simulink model "new_inkine_2020"  (R2022b)
settings: Solver=FixedStepAuto  StartTime=0.0  StopTime=250  FixedStep=0.001  RelTol=1e-3
PreLoadFcn:
  | parameters_new;
InitFcn:
  | parameters_new;
(part 1 of 3)
settings Model: Creator=Yubin  LastModifiedBy=峰
settings SolverCC: AlgebraicLoopSolver=TrustRegion
settings ConfigComp: PLC_OutputDir=D:\Documents\Visual Studio 2015\Projects  PLC_TargetIDE=twincat3  PLC_MultiTBSigbuilderTimeRange=off  PLC_FoldFBCallOutputVar=off  PLC_InlineEnumCastFunction=off

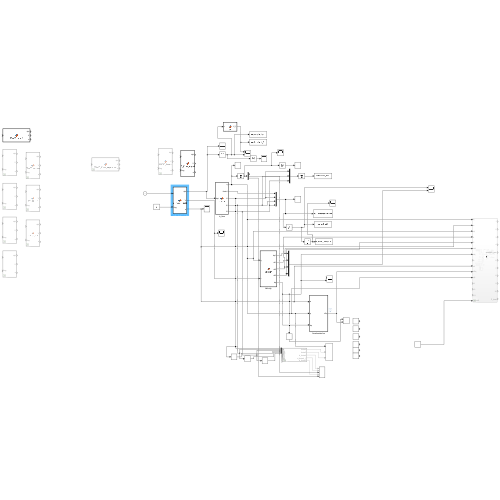
[thumbnail: Simulink's stored preview of the top-level diagram]
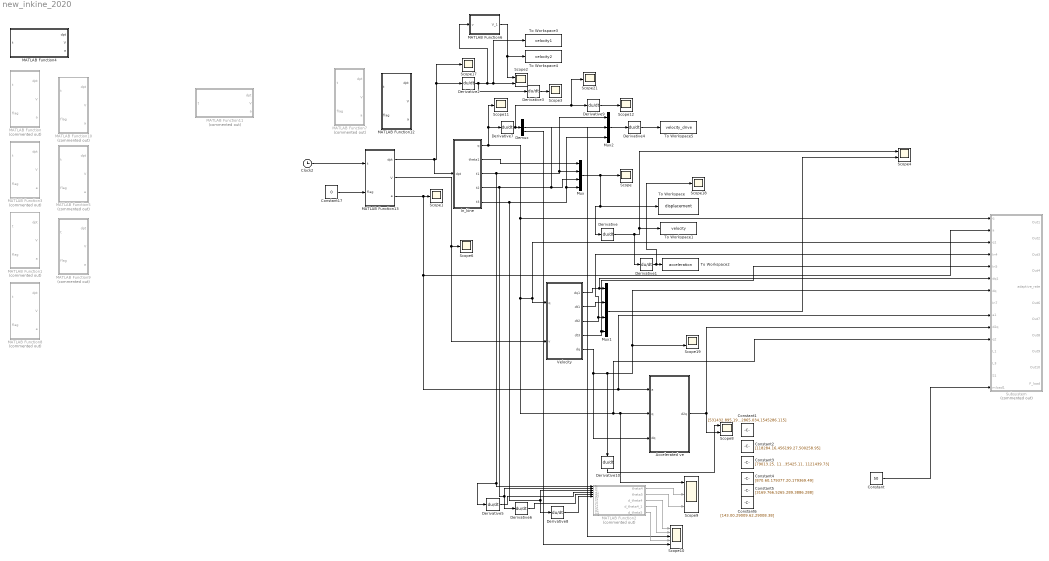
== system new_inkine_2020 ==
  Accelerated ve : MATLAB Function  TreatAsAtomicUnit=on
  Clock2 : Clock
      settings: Decimation=50
  Constant : Constant  Value=50
  Constant1 : Constant  Value=[531432.895,1962865.034,1545286.115]
  Constant17 : Constant  Value=0
  Constant2 : Constant  Value=[118284.16,456199.27,500258.95]
  Constant3 : Constant  Value=[79013.25, 1135425.11, 1121439.73]
  Constant4 : Constant  Value=[870.60,179377.20,179369.49]
  Constant5 : Constant  Value=[3169.766,5265.289,3886.288]
  Constant6 : Constant  Value=[143.00,29009.62,29008.38]
  Demux : Demux  Outputs=3
  Derivative{,1..10} (11 alike) : Derivative
  In_kine : MATLAB Function  TreatAsAtomicUnit=on
  MATLAB Function : MATLAB Function  Commented=on  TreatAsAtomicUnit=on
  MATLAB Function1 : MATLAB Function  Commented=on  TreatAsAtomicUnit=on
  MATLAB Function10 : MATLAB Function  Commented=on  TreatAsAtomicUnit=on
  MATLAB Function11 : MATLAB Function  Commented=on  TreatAsAtomicUnit=on
  MATLAB Function12 : MATLAB Function  TreatAsAtomicUnit=on
  MATLAB Function13 : MATLAB Function  TreatAsAtomicUnit=on
  MATLAB Function2 : MATLAB Function  Commented=on  TreatAsAtomicUnit=on
  MATLAB Function3 : MATLAB Function  Commented=on  TreatAsAtomicUnit=on
  MATLAB Function4 : MATLAB Function  TreatAsAtomicUnit=on
  MATLAB Function5 : MATLAB Function  Commented=on  TreatAsAtomicUnit=on
  MATLAB Function6 : MATLAB Function  TreatAsAtomicUnit=on
  MATLAB Function7 : MATLAB Function  Commented=on  TreatAsAtomicUnit=on
  MATLAB Function8 : MATLAB Function  Commented=on  TreatAsAtomicUnit=on
  MATLAB Function9 : MATLAB Function  Commented=on  TreatAsAtomicUnit=on
  Mux : Mux
  Mux1 : Mux
  Mux2 : Mux  Inputs=3
  Scope{,1,3,6,11..12,17..18,21} (9 alike) : Scope
  Scope10 : Scope  NumInputPorts=5
  Scope{2,4,8,19} (4 alike) : Scope  NumInputPorts=2
  Scope9 : Scope  NumInputPorts=3
  Subsystem : Subsystem  Commented=on
  To Workspace : ToWorkspace  VariableName=displacement  SaveFormat=Timeseries  SampleTime=-1
  To Workspace1 : ToWorkspace  VariableName=velocity  SaveFormat=Timeseries  SampleTime=-1
  To Workspace2 : ToWorkspace  VariableName=acceleration  SaveFormat=Timeseries  SampleTime=-1
  To Workspace3 : ToWorkspace  VariableName=velocity1  SampleTime=-1
      settings: Save2DSignal=2-D array (concatenate along first dimension)
  To Workspace4 : ToWorkspace  VariableName=velocity2  SampleTime=-1
      settings: Save2DSignal=2-D array (concatenate along first dimension)
  To Workspace5 : ToWorkspace  VariableName=velocity_drive  SampleTime=-1
      settings: Save2DSignal=2-D array (concatenate along first dimension)
  Velocity : MATLAB Function  TreatAsAtomicUnit=on
  wires:
  In_kine/2(theta1) -> Mux/1
  Clock2/1 -> MATLAB Function13/1(t)
  Derivative/1 -> Scope4/1, To Workspace1/1, Derivative1/1
  Derivative1/1 -> Scope18/1, To Workspace2/1
  MATLAB Function13/1(dpt) -> In_kine/1(dpt), Scope17/1, Derivative2/1
  Derivative3/1 -> Scope3/1
  MATLAB Function13/3(a) -> Subsystem/9(a1), Accelerated ve/1(a), Subsystem/2(a), Scope1/1
  Velocity/1(dq1) -> Subsystem/6(dq1), Mux1/1
  Velocity/2(dt1) -> Mux1/2
  Velocity/3(dt2) -> Mux1/3, Subsystem/4(In4)
  Velocity/4(dt3) -> Subsystem/5(In5), Mux1/4
  Mux1/1 -> Scope4/2
  MATLAB Function13/2(V) -> Velocity/2(v), Scope6/1
  Velocity/5(dq) -> Accelerated ve/3(dq), Subsystem/7(dq), Scope19/2, Derivative10/1
  Accelerated ve/1(d2q) -> Subsystem/10(d2q), Scope8/2
  MATLAB Function2/1(theta4) -> Scope9/2
  MATLAB Function2/2(theta5) -> Scope9/3
  MATLAB Function2/3(d_theta4) -> Scope10/1
  Demux/2 -> Scope10/3
  MATLAB Function2/5(d_theta5) -> Scope10/4
  Derivative7/1 -> Scope21/1, Derivative9/1, Demux/1
  Demux/3 -> Scope10/5
  MATLAB Function2/4(d_theta4_1) -> Scope10/2
  Derivative5/1 -> MATLAB Function2/4(dt1)
  In_kine/4(t2) -> Derivative6/1, MATLAB Function2/2(t2), Mux/3, Mux2/2
  In_kine/5(t3) -> Derivative8/1, MATLAB Function2/3(t3), Mux2/3, Mux/4
  Derivative6/1 -> MATLAB Function2/5(dt2)
  Derivative8/1 -> MATLAB Function2/6(dt3)
  Constant17/1 -> MATLAB Function13/2(flag)
  Derivative9/1 -> Scope12/1
  Mux/1 -> Scope/1, Derivative/1, To Workspace/1
  Derivative10/1 -> Scope8/1
  In_kine/1(q) -> Scope11/1, Derivative7/1, Subsystem/1(q), Velocity/1(q), Subsystem/3(q1), Subsystem/11(q2), Scope9/1, Accelerated ve/2(q)
  MATLAB Function6/1(V_1) -> To Workspace4/1, Scope2/1
  Constant/1 -> Subsystem/15(mload1)
  Derivative2/1 -> Derivative3/1, MATLAB Function6/1(v), Scope2/2, To Workspace3/1
  In_kine/3(t1) -> Derivative5/1, MATLAB Function2/1(t1), Mux/2, Mux2/1
  Mux2/1 -> Derivative4/1
  Derivative4/1 -> To Workspace5/1

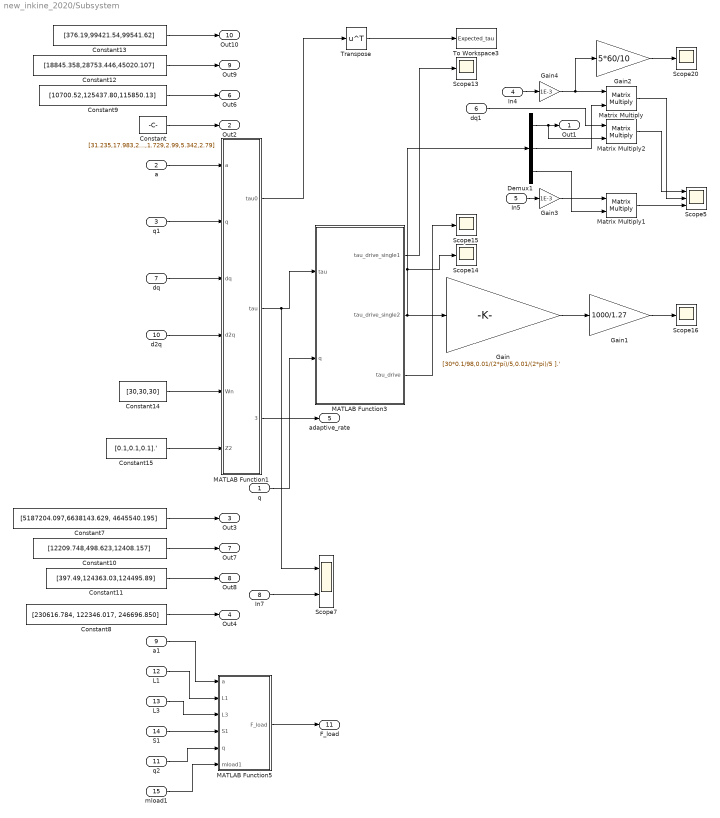
== system new_inkine_2020/Subsystem ==
  q : Inport
  a : Inport  Port=2
  q1 : Inport  Port=3
  In4 : Inport  Port=4
  In5 : Inport  Port=5
  dq1 : Inport  Port=6
  dq : Inport  Port=7
  In7 : Inport  Port=8
  a1 : Inport  Port=9
  d2q : Inport  Port=10
  q2 : Inport  Port=11
  L1 : Inport  Port=12
  L3 : Inport  Port=13
  S1 : Inport  Port=14
  mload1 : Inport  Port=15
  Constant : Constant  Value=[31.235,17.983,21.8,5.16,2.248,2.248,1.73,1.73,121.413,13.425,3.54,1.729,2.99,5.342,2.79]
  Constant10 : Constant  Value=[12209.748,498.623,12408.157]
  Constant11 : Constant  Value=[397.49,124363.03,124495.89]
  Constant12 : Constant  Value=[18845.358,28753.446,45020.107]
  Constant13 : Constant  Value=[376.19,99421.54,99541.62]
  Constant14 : Constant  Value=[30,30,30]
  Constant15 : Constant  Value=[0.1,0.1,0.1].'
  Constant7 : Constant  Value=[5187204.097,6638143.629, 4645540.195]
  Constant8 : Constant  Value=[230616.784, 122346.017, 246696.850]
  Constant9 : Constant  Value=[10700.52,125437.80,115850.13]
  Demux1 : Demux  Outputs=3
  Gain : Gain  Gain=[30*0.1/98,0.01/(2*pi)/5,0.01/(2*pi)/5 ].'
  Gain1 : Gain  Gain=1000/1.27
  Gain2 : Gain  Gain=5*60/10
  Gain3 : Gain  Gain=1E-3
  Gain4 : Gain  Gain=1E-3
  MATLAB Function1 : MATLAB Function  TreatAsAtomicUnit=on
  MATLAB Function3 : MATLAB Function  TreatAsAtomicUnit=on
  MATLAB Function5 : MATLAB Function  TreatAsAtomicUnit=on
  Matrix Multiply : Product  Multiplication=Matrix(*)
  Matrix Multiply1 : Product  Multiplication=Matrix(*)
  Matrix Multiply2 : Product  Multiplication=Matrix(*)
  Scope{13..16,20} (5 alike) : Scope
  Scope5 : Scope  NumInputPorts=3
  Scope7 : Scope  NumInputPorts=2
  To Workspace3 : ToWorkspace  VariableName=Expected_tau  SampleTime=-1
      settings: Save2DSignal=2-D array (concatenate along first dimension)
  Transpose : Math  Operator=transpose
  Out1 : Outport
  Out2 : Outport  Port=2
  Out3 : Outport  Port=3
  Out4 : Outport  Port=4
  adaptive_rate : Outport  Port=5
  Out6 : Outport  Port=6
  Out7 : Outport  Port=7
  Out8 : Outport  Port=8
  Out9 : Outport  Port=9
  Out10 : Outport  Port=10
  F_load : Outport  Port=11
  wires:
  Constant/1 -> Out2/1
  d2q/1 -> MATLAB Function1/4(d2q)
  Demux1/1 -> Matrix Multiply2/2, Out1/1
  L1/1 -> MATLAB Function5/2(L1)
  Constant13/1 -> Out10/1
  q1/1 -> MATLAB Function1/2(q)
  Constant9/1 -> Out6/1
  Constant12/1 -> Out9/1
  a/1 -> MATLAB Function1/1(a)
  dq/1 -> MATLAB Function1/3(dq)
  Constant15/1 -> MATLAB Function1/6(Z2)
  Constant14/1 -> MATLAB Function1/5(Wn)
  Constant7/1 -> Out3/1
  Constant10/1 -> Out7/1
  In7/1 -> Scope7/2
  Constant11/1 -> Out8/1
  In5/1 -> Gain3/1
  S1/1 -> MATLAB Function5/4(S1)
  Constant8/1 -> Out4/1
  q/1 -> MATLAB Function3/2(q)
  a1/1 -> MATLAB Function5/1(a)
  In4/1 -> Gain4/1
  L3/1 -> MATLAB Function5/3(L3)
  q2/1 -> MATLAB Function5/5(q)
  mload1/1 -> MATLAB Function5/6(mload1)
  MATLAB Function1/1(tau0) -> Transpose/1
  MATLAB Function1/2(tau) -> Scope7/1, MATLAB Function3/1(tau)
  Gain/1 -> Gain1/1
  MATLAB Function1/3(adaptive_rate) -> adaptive_rate/1
  MATLAB Function5/1(F_load) -> F_load/1
  Transpose/1 -> To Workspace3/1
  MATLAB Function3/3(tau_drive) -> Scope15/1
  MATLAB Function3/1(tau_drive_single1) -> Scope13/1
  MATLAB Function3/2(tau_drive_single2) -> Scope14/1, Demux1/1, Gain/1
  Demux1/2 -> Matrix Multiply/2
  Gain2/1 -> Scope20/1
  Demux1/3 -> Matrix Multiply1/2
  Matrix Multiply/1 -> Scope5/2
  Matrix Multiply1/1 -> Scope5/3
  Gain1/1 -> Scope16/1
  dq1/1 -> Matrix Multiply2/1
  Matrix Multiply2/1 -> Scope5/1
  Gain3/1 -> Matrix Multiply1/1
  Gain4/1 -> Gain2/1, Matrix Multiply/1

== matlab function new_inkine_2020/MATLAB Function2 ==
  data: t1 input; theta4 output; t2 input; theta5 output; t3 input; dt1 input; dt2 input; d_theta4 output; d_theta4_1 output; dt3 input; d_theta5 output; R1 input; R2 input; Le input; K1 input; K2 input; M1 input; M2 input; TT1 input; TT2 input
function [theta4,theta5,d_theta4,d_theta4_1,d_theta5]  =kinematics(t1,t2,t3,dt1,dt2,dt3,...
    R1,R2,Le,K1,K2,M1,M2,TT1,TT2)
% coder.extrinsic('evalin');
% R1=0;R2=0;Le=0;K1=0;K2=0;M1=0;M2=0;T1=0;T2=0;
% R1=evalin('base','R1');Le=evalin('base','Le');R2=evalin('base','R2');
% K1=evalin('base','K1');K2=evalin('base','K2');M1=evalin('base','M1');M2=evalin('base','M2');T1=evalin('base','T1');T2=evalin('base','T2');
% -X1-T1=t1   -y1-T2=t2
x1=-(t1+TT1);y1=-(t2+TT2);
theta6=5*pi/6;theta7=-pi/6;
%广义坐标位置的求取
theta2=asin((Le^2-R1^2-K1^2-x1^2)/(-2*R1*sqrt(x1^2+K1^2)))-atan(x1/K1);
theta2_1=-asin((Le^2-R1^2-K2^2-y1^2)/(-2*R1*sqrt(y1^2+K2^2)))-atan(K2/y1);
theta3=asin((R2^2+M1^2+M2^2-t3^2)/(2*R2*sqrt(M1^2+M2^2)))-atan(M1/M2);

theta4=theta6-theta2;theta4_1=theta6-theta2_1;theta5=theta7-theta3;
%广义坐标速度的求取
d_theta4=((x1*(K1^2 + Le^2 - R1^2 + x1^2))/...
    (2*R1*sqrt(1 - (K1^2 - Le^2 + R1^2 + x1^2)^2/(4*R1^2*(K1^2 + x1^2)))*(K1^2 + x1^2)^(3/2)) ...
    - K1/(K1^2 + x1^2))*dt1;
d_theta4_1=(K2/(K2^2 + y1^2) -...
    (y1*(K2^2 + Le^2 - R1^2 + y1^2))/...
    (2*R1*sqrt(1 - (K2^2 - Le^2 + R1^2 + y1^2)^2/(4*R1^2*(K2^2 + y1^2)))*(K2^2 + y1^2)^(3/2)))*dt2;
d_theta5=t3/(R2*sqrt(1 - (M1^2 + M2^2 + R2^2 - t3^2)^2/(4*R2^2*(M1^2 + M2^2)))*sqrt(M1^2 + M2^2))*dt3;

== matlab function new_inkine_2020/MATLAB Function ==
  data: t input; dpt output; V output; a output; flag input
function [dpt,V,a] = TRACE(t,flag)%轨迹规划
if flag==1
K_1=0;KV_1=0;Ka_1=0;
[K_2,KV_2,Ka_2]=polynomial_v((t-2),1, 0,0,0, 125,180,10);%2-3
[K_3,KV_3,Ka_3]=polynomial_v((t-3),0.5, 125,180,10, 225,200,-60);%3-3.5
[K_4,KV_4,Ka_4]=polynomial_v((t-3.5),0.5, 225,200,-60, 325,200,120);%3.5-4
[K_5,KV_5,Ka_5]=polynomial_v((t-4),1, 325,200,120, 475, 0,0);%4-5
X=K_1.*(t>=0&t<2)+K_2.*(t>=2&t<3)+K_3.*(t>=3&t<3.5)+K_4.*(t>=3.5&t<4)+K_5.*(t>=4&t<=5);
VX=KV_1.*(t>=0&t<2)+KV_2.*(t>=2&t<3)+KV_3.*(t>=3&t<3.5)+KV_4.*(t>=3.5&t<4)+KV_5.*(t>=4&t<=5);
aX=Ka_1.*(t>=0&t<2)+Ka_2.*(t>=2&t<3)+Ka_3.*(t>=3&t<3.5)+Ka_4.*(t>=3.5&t<4)+Ka_5.*(t>=4&t<=5);

S_1=225;SV_1=0;Sa_1=0;
[S_2,SV_2,Sa_2]=polynomial_v((t-2),1, 225,0,0, 90,-120,210);%2-3s
[S_3,SV_3,Sa_3]=polynomial_v((t-3),0.5, 90,-120,210, 45,-75,45);%3-3.5s
[S_4,SV_4,Sa_4]=polynomial_v((t-3.5),0.5, 45,-75,45, 20,-36,10);%3.5-4s
[S_5,SV_5,Sa_5]=polynomial_v((t-4),1, 20,-36,10, 0, 0,0);%4-5s
Y=S_1.*(t>=0&t<2)+S_2.*(t>=2&t<3)+S_3.*(t>=3&t<3.5)+S_4.*(t>=3.5&t<4)+S_5.*(t>=4&t<=5);
VY=SV_1.*(t>=0&t<2)+SV_2.*(t>=2&t<3)+SV_3.*(t>=3&t<3.5)+SV_4.*(t>=3.5&t<4)+SV_5.*(t>=4&t<=5);
aY=Sa_1.*(t>=0&t<2)+Sa_2.*(t>=2&t<3)+Sa_3.*(t>=3&t<3.5)+Sa_4.*(t>=3.5&t<4)+Sa_5.*(t>=4&t<=5);

[Z_1,ZV_1,Za_1]=polynomial_v(t,2,1300,0,0,1000,0,0);
Z_2=1000;ZV_2=0;Za_2=0;
Z=Z_1.*(t>=0&t<2)+Z_2.*(t>=2&t<=5);
VZ=ZV_1.*(t>=0&t<2)+ZV_2.*(t>=2&t<=5);
aZ=Za_1.*(t>=0&t<2)+Za_2.*(t>=2&t<=5);

dpt=[X,Y,Z];V=[VX,VY,VZ]; a=[aX,aY,aZ].';


elseif flag==2
    
K_1=0;KV_1=0;Ka_1=0;
[K_2,KV_2,Ka_2]=polynomial_v((t-4),2, 0,0,0, 125,90,10);%4-6
[K_3,KV_3,Ka_3]=polynomial_v((t-6),1, 125,90,10, 225,100,0);%6-7
[K_4,KV_4,Ka_4]=polynomial_v((t-7),1, 225,100,0, 325,100,20);%7-8
[K_5,KV_5,Ka_5]=polynomial_v((t-8),2, 325,100,20, 475, 0,0);%8-10
X=K_1.*(t>=0&t<4)+K_2.*(t>=4&t<6)+K_3.*(t>=6&t<7)+K_4.*(t>=7&t<8)+K_5.*(t>=8&t<=10);
VX=KV_1.*(t>=0&t<4)+KV_2.*(t>=4&t<6)+KV_3.*(t>=6&t<7)+KV_4.*(t>=7&t<8)+KV_5.*(t>=8&t<=10);
aX=Ka_1.*(t>=0&t<4)+Ka_2.*(t>=4&t<6)+Ka_3.*(t>=6&t<7)+Ka_4.*(t>=7&t<8)+Ka_5.*(t>=8&t<=10);


S_1=225;SV_1=0;Sa_1=0;
[S_2,SV_2,Sa_2]=polynomial_v((t-4),2, 225,0,0, 90,-60,60);%4-6s
[S_3,SV_3,Sa_3]=polynomial_v((t-6),1, 90,-60,60, 45,-35,20);%6-7s
[S_4,SV_4,Sa_4]=polynomial_v((t-7),1, 45,-35,20, 20,-18,10);%7-8s
[S_5,SV_5,Sa_5]=polynomial_v((t-8),2, 20,-18,10, 0, 0,0);%8-10s
Y=S_1.*(t>=0&t<4)+S_2.*(t>=4&t<6)+S_3.*(t>=6&t<7)+S_4.*(t>=7&t<8)+S_5.*(t>=8&t<=10);
VY=SV_1.*(t>=0&t<4)+SV_2.*(t>=4&t<6)+SV_3.*(t>=6&t<7)+SV_4.*(t>=7&t<8)+SV_5.*(t>=8&t<=10);
aY=Sa_1.*(t>=0&t<4)+Sa_2.*(t>=4&t<6)+Sa_3.*(t>=6&t<7)+Sa_4.*(t>=7&t<8)+Sa_5.*(t>=8&t<=10);

[Z_1,ZV_1,Za_1]=polynomial_v(t,4,1300,0,0,1000,0,0);
Z_2=1000;ZV_2=0;Za_2=0;
Z=Z_1.*(t>=0&t<4)+Z_2.*(t>=4&t<=10);
VZ=ZV_1.*(t>=0&t<4)+ZV_2.*(t>=4&t<=10);
aZ=Za_1.*(t>=0&t<4)+Za_2.*(t>=4&t<=10);

dpt=[X,Y,Z];V=[VX,VY,VZ]; a=[aX,aY,aZ].';

else
K_1=0;KV_1=0;Ka_1=0;
[K_2,KV_2,Ka_2]=polynomial_v((t-6),3, 0,0,0, 125,60,5);%6-9
[K_3,KV_3,Ka_3]=polynomial_v((t-9),1.5, 125,60,5, 225,65,0);%9-10.5
[K_4,KV_4,Ka_4]=polynomial_v((t-10.5),1.5, 225,65,0, 325,65,7);%10.5-12
[K_5,KV_5,Ka_5]=polynomial_v((t-12),3, 325,65,7, 475, 0,0);%12-15
X=K_1.*(t>=0&t<6)+K_2.*(t>=6&t<9)+K_3.*(t>=9&t<10.5)+K_4.*(t>=10.5&t<12)+K_5.*(t>=12&t<=15);
VX=KV_1.*(t>=0&t<6)+KV_2.*(t>=6&t<9)+KV_3.*(t>=9&t<10.5)+KV_4.*(t>=10.5&t<12)+KV_5.*(t>=12&t<=15);
aX=Ka_1.*(t>=0&t<6)+Ka_2.*(t>=6&t<9)+Ka_3.*(t>=9&t<10.5)+Ka_4.*(t>=10.5&t<12)+Ka_5.*(t>=12&t<=15);


S_1=225;SV_1=0;Sa_1=0;
[S_2,SV_2,Sa_2]=polynomial_v((t-6),3, 225,0,0, 90,-40,20);%4-6s
[S_3,SV_3,Sa_3]=polynomial_v((t-9),1.5, 90,-40,20, 45,-24,5);%6-7s
[S_4,SV_4,Sa_4]=polynomial_v((t-10.5),1.5, 45,-24,5, 20,-12,5);%7-8s
[S_5,SV_5,Sa_5]=polynomial_v((t-12),3, 20,-12,5, 0, 0,0);%8-10s
Y=S_1.*(t>=0&t<6)+S_2.*(t>=6&t<9)+S_3.*(t>=9&t<10.5)+S_4.*(t>=10.5&t<12)+S_5.*(t>=12&t<=15);
VY=SV_1.*(t>=0&t<6)+SV_2.*(t>=6&t<9)+SV_3.*(t>=9&t<10.5)+SV_4.*(t>=10.5&t<12)+SV_5.*(t>=12&t<=15);
aY=Sa_1.*(t>=0&t<6)+Sa_2.*(t>=6&t<9)+Sa_3.*(t>=9&t<10.5)+Sa_4.*(t>=10.5&t<12)+Sa_5.*(t>=12&t<=15);

[Z_1,ZV_1,Za_1]=polynomial_v(t,6,1300,0,0,1000,0,0);
Z_2=1000;ZV_2=0;Za_2=0;
Z=Z_1.*(t>=0&t<6)+Z_2.*(t>=6&t<=15);
VZ=ZV_1.*(t>=0&t<6)+ZV_2.*(t>=6&t<=15);
aZ=Za_1.*(t>=0&t<6)+Za_2.*(t>=6&t<=15);

dpt=[X,Y,Z];V=[VX,VY,VZ]; a=[aX,aY,aZ].';
end
end

== matlab function new_inkine_2020/Subsystem/MATLAB Function3 ==
  data: tau input; q input; tau_drive_single1 output; tau_drive_single2 output; tau_drive output
function [tau_drive_single1,tau_drive_single2,tau_drive] = Tau_distribution(tau,q)
L1=0;L3=0;S1=0;R1=0;R2=0;Le=0;K1=0;K2=0;M1=0;M2=0;
coder.extrinsic('evalin');
L1=evalin('base','L1');L3=evalin('base','L3');S1=evalin('base','S1');R1=evalin('base','R1');Le=evalin('base','Le');R2=evalin('base','R2');
K1=evalin('base','K1');K2=evalin('base','K2');M1=evalin('base','M1');M2=evalin('base','M2');
S1=82;L1=600;L3=550;M1=312.5;M2=140.5;R2=318;
R1=200;Le=414;K1=270;L2=215;L11=532;S3=150;S4=180;
L7=Le;L8=Le;
Lc14=100.63;Lc14y=49.13;
LC1y=7.69;LC2=-38.71;LC2y=-48.68;LC3=167.99;
L9=sqrt(4.13^2+2.45^2);Lcx10=-13.9;
Ls5=268.5;Ls6=-242.5;Ls11=189; Ls13=189; %偏置
theta6=5*pi/6;theta7=-pi/6;
theta4=q(2);theta5=q(3);
theta2=theta6-theta4;theta3=theta7-theta5;
phi1=asin((K1-R1*sin(theta2))/L7);
phi2=acos((K2-R1*cos(theta2))/L8);

n=sqrt((M1 - R2*cos(theta3))^2 + (M2 - R2*sin(theta3))^2);
f1=(-R1*sin(theta2)-R1*cos(theta2)*tan(phi1))*10^(-3);
f2=(R1*cos(theta2)+(R1*sin(theta2))/tan(phi2))*10^(-3);
g3=(-R2*(M1*sin(theta3)-M2*cos(theta3))/n)*10^(-3);
D=[1 0 0 0;0 f1 f2 0;0 0 0 g3];
D1=D.'/(D*D.');
D01=[1 0 0 ;0 f1 0;0 0 g3];
D02=[1 0 0 ;0 f2 0;0 0 g3];
tau_drive=D1*tau;
tau_drive_single1=inv(D01)*tau;
tau_drive_single2=inv(D02)*tau;

== matlab function new_inkine_2020/MATLAB Function4 ==
  data: t input; dpt output; V output; a output
function [dpt,V,a] = TRACE_slow2(t)
K_1=0;KV_1=0;Ka_1=0;
[K_2,KV_2,Ka_2]=polynomial_v((t-6),3, 0,0,0, 125,60,5);%6-9
[K_3,KV_3,Ka_3]=polynomial_v((t-9),1.5, 125,60,5, 225,65,0);%9-10.5
[K_4,KV_4,Ka_4]=polynomial_v((t-10.5),1.5, 225,65,0, 325,65,7);%10.5-12
[K_5,KV_5,Ka_5]=polynomial_v((t-12),3, 325,65,7, 475, 0,0);%12-15
X=K_1.*(t>=0&t<6)+K_2.*(t>=6&t<9)+K_3.*(t>=9&t<10.5)+K_4.*(t>=10.5&t<12)+K_5.*(t>=12&t<=15);
VX=KV_1.*(t>=0&t<6)+KV_2.*(t>=6&t<9)+KV_3.*(t>=9&t<10.5)+KV_4.*(t>=10.5&t<12)+KV_5.*(t>=12&t<=15);
aX=Ka_1.*(t>=0&t<6)+Ka_2.*(t>=6&t<9)+Ka_3.*(t>=9&t<10.5)+Ka_4.*(t>=10.5&t<12)+Ka_5.*(t>=12&t<=15);


S_1=225;SV_1=0;Sa_1=0;
[S_2,SV_2,Sa_2]=polynomial_v((t-6),3, 225,0,0, 90,-40,20);%4-6s
[S_3,SV_3,Sa_3]=polynomial_v((t-9),1.5, 90,-40,20, 45,-24,5);%6-7s
[S_4,SV_4,Sa_4]=polynomial_v((t-10.5),1.5, 45,-24,5, 20,-12,5);%7-8s
[S_5,SV_5,Sa_5]=polynomial_v((t-12),3, 20,-12,5, 0, 0,0);%8-10s
Y=S_1.*(t>=0&t<6)+S_2.*(t>=6&t<9)+S_3.*(t>=9&t<10.5)+S_4.*(t>=10.5&t<12)+S_5.*(t>=12&t<=15);
VY=SV_1.*(t>=0&t<6)+SV_2.*(t>=6&t<9)+SV_3.*(t>=9&t<10.5)+SV_4.*(t>=10.5&t<12)+SV_5.*(t>=12&t<=15);
aY=Sa_1.*(t>=0&t<6)+Sa_2.*(t>=6&t<9)+Sa_3.*(t>=9&t<10.5)+Sa_4.*(t>=10.5&t<12)+Sa_5.*(t>=12&t<=15);

[Z_1,ZV_1,Za_1]=polynomial_v(t,6,1300,0,0,1000,0,0);
Z_2=1000;ZV_2=0;Za_2=0;
Z=Z_1.*(t>=0&t<6)+Z_2.*(t>=6&t<=15);
VZ=ZV_1.*(t>=0&t<6)+ZV_2.*(t>=6&t<=15);
aZ=Za_1.*(t>=0&t<6)+Za_2.*(t>=6&t<=15);

dpt=[X,Y,Z];V=[VX,VY,VZ]; a=[aX,aY,aZ].';
end

== matlab function new_inkine_2020/Subsystem/MATLAB Function5 ==
  data: a input; L1 input; F_load output; L3 input; S1 input; q input; mload1 input
function F_load = T_load(a,L1,L3,S1,q,mload1)
g=9806.65;
theta1=q(1);theta4=q(2);theta5=q(3);
jacobian=[-sin(theta1)*(L1*cos(theta4)+L3*cos(theta5)-S1) -L1*cos(theta1)*sin(theta4) -L3*cos(theta1)*sin(theta5) ;
    cos(theta1)*(L1*cos(theta4)+L3*cos(theta5)-S1) -L1*sin(theta1)*sin(theta4) -L3*sin(theta1)*sin(theta5) ;
    0 L1*cos(theta4) L3*cos(theta5) ];
G_load=[0,0,mload1*g].';Fa_load=mload1*a;
F_load=-jacobian.'*(-Fa_load+G_load);

== matlab function new_inkine_2020/MATLAB Function6 ==
  data: v input; V_1 output
function V_1 = fcn(v)
 V_1=norm(v);

== matlab function new_inkine_2020/MATLAB Function7 ==
  data: t input; dpt output; V output; a output; flag input
function [dpt,V,a] = TRACE_Access(t,flag)%轨迹规划
 dpt = zeros(1,3); % 明确输出是1x3向量
    V = zeros(1,3);
    a = zeros(1,3);
if flag==1
%x轴
 [X,VX,aX]=S_xing(125, 475, 0, 0, 20, 20, 30,t);
 [Y,VY,aY]=S_xing(0, 90, 0, 0, 20, 20, 30,t);
 [Z,VZ,aZ]=S_xing(980, 1300, 0, 0, 10, 10, 30,t);
%      [X,Y,Z]=S_xing(475, 0, 0, 0, 10, 10, 1);
%      [VX,VY,VZ]=S_xing(0, 0, 0, 0, 1, 1, 1);
%      [aX,aY,aZ]=S_xing(980, 980, 0, 0, 1, 1, 1);
     dpt=[X,Y,Z];V=[VX,VY,VZ]; a=[aX,aY,aZ];
  else
    

[K_1,KV_1,Ka_1]=polynomial_v(t,2, 475, 0,0, 325,-90,20);%4-6
[K_2,KV_2,Ka_2]=polynomial_v((t-2),1, 325,-90,20, 225,-120,-10);%6-7
[K_3,KV_3,Ka_3]=polynomial_v((t-3),1, 225,-120,-10, 125,-100,-20);%7-8
[K_4,KV_4,Ka_4]=polynomial_v((t-4),2, 125,-100,-20 , 0,0,0);%8-10
K_5=0;KV_5=0;Ka_5=0;
X=K_1.*(t>=0&t<2)+K_2.*(t>=2&t<3)+K_3.*(t>=3&t<4)+K_4.*(t>=4&t<6)+K_5.*(t>=6&t<=10);
VX=KV_1.*(t>=0&t<2)+KV_2.*(t>=2&t<3)+KV_3.*(t>=3&t<4)+KV_4.*(t>=4&t<6)+KV_5.*(t>=6&t<=10);
aX=Ka_1.*(t>=0&t<2)+Ka_2.*(t>=2&t<3)+Ka_3.*(t>=3&t<4)+Ka_4.*(t>=4&t<6)+Ka_5.*(t>=6&t<=10);



[S_1,SV_1,Sa_1]=polynomial_v(t,2, 0,0,0, 20,15,15);%4-6s
[S_2,SV_2,Sa_2]=polynomial_v((t-2),1, 20,15,15, 45,30,-10);%6-7s
[S_3,SV_3,Sa_3]=polynomial_v((t-3),1, 45,30,-10, 90,80,80);%7-8s
[S_4,SV_4,Sa_4]=polynomial_v((t-4),2, 90,80,80, 225,0,0);%8-10s
S_5=225;SV_5=0;Sa_5=0;
Y=S_1.*(t>=0&t<2)+S_2.*(t>=2&t<3)+S_3.*(t>=3&t<4)+S_4.*(t>=4&t<6)+S_5.*(t>=6&t<=10);
VY=SV_1.*(t>=0&t<2)+SV_2.*(t>=2&t<3)+SV_3.*(t>=3&t<4)+SV_4.*(t>=4&t<6)+SV_5.*(t>=6&t<=10);
aY=Sa_1.*(t>=0&t<2)+Sa_2.*(t>=2&t<3)+Sa_3.*(t>=3&t<4)+Sa_4.*(t>=4&t<6)+Sa_5.*(t>=6&t<=10);

[Z_1,ZV_1,Za_1]=polynomial_v((t-6),4,980,0,0,1300,0,0);
Z_2=980;ZV_2=0;Za_2=0;
Z=Z_2.*(t>=0&t<6)+Z_1.*(t>=6&t<=10);
VZ=ZV_2.*(t>=0&t<6)+ZV_1.*(t>=6&t<=10);
aZ=Za_2.*(t>=0&t<6)+Za_1.*(t>=6&t<=10);

dpt=[X,Y,Z];V=[VX,VY,VZ]; a=[aX,aY,aZ];



end
end

== matlab function new_inkine_2020/MATLAB Function1 ==
  data: t input; dpt output; V output; a output; flag input
function [dpt,V,a] = TRACE_NEW(t,flag)%轨迹规划
if flag==1
[K_1,KV_1,Ka_1]=polynomial_v(t,1, 475, 0,0, 325,-200,60);%0-1
[K_2,KV_2,Ka_2]=polynomial_v((t-1),0.5, 325,-200,60, 225,-200,-20);%1-1.5
[K_3,KV_3,Ka_3]=polynomial_v((t-1.5),0.5, 225,-200,-20, 125,-180,-0);%1.5-2
[K_4,KV_4,Ka_4]=polynomial_v((t-2),1, 125,-180,-10, 0,0,0);%2-3
K_5=0;KV_5=0;Ka_5=0;
X=K_1.*(t>=0&t<1)+K_2.*(t>=1&t<1.5)+K_3.*(t>=1.5&t<2)+K_4.*(t>=2&t<3)+K_5.*(t>=3&t<=5);
VX=KV_1.*(t>=0&t<1)+KV_2.*(t>=1&t<1.5)+KV_3.*(t>=1.5&t<2)+KV_4.*(t>=2&t<3)+KV_5.*(t>=3&t<=5);
aX=Ka_1.*(t>=0&t<1)+Ka_2.*(t>=1&t<1.5)+Ka_3.*(t>=1.5&t<2)+Ka_4.*(t>=2&t<3)+Ka_5.*(t>=3&t<=5);

[S_1,SV_1,Sa_1]=polynomial_v(t,1, 0,0,0, 20,36,-10);%0-1s
[S_2,SV_2,Sa_2]=polynomial_v((t-1),0.5, 20,36,-10, 45,75,25);%1-1.5s
[S_3,SV_3,Sa_3]=polynomial_v((t-1.5),0.5, 45,75,25, 90,150,300);%1.5-2s
[S_4,SV_4,Sa_4]=polynomial_v((t-2),1, 90,150,300, 225,0,0);%2-3s
S_5=225;SV_5=0;Sa_5=0;

Y=S_1.*(t>=0&t<1)+S_2.*(t>=1&t<1.5)+S_3.*(t>=1.5&t<2)+S_4.*(t>=2&t<3)+S_5.*(t>=3&t<=5);
VY=SV_1.*(t>=0&t<1)+SV_2.*(t>=1&t<1.5)+SV_3.*(t>=1.5&t<2)+SV_4.*(t>=2&t<3)+SV_5.*(t>=3&t<=5);
aY=Sa_1.*(t>=0&t<1)+Sa_2.*(t>=1&t<1.5)+Sa_3.*(t>=1.5&t<2)+Sa_4.*(t>=2&t<3)+Sa_5.*(t>=3&t<=5);

[Z_1,ZV_1,Za_1]=polynomial_v((t-3),2,980,0,0,1300,0,0);
Z_2=980;ZV_2=0;Za_2=0;
Z=Z_2.*(t>=0&t<3)+Z_1.*(t>=3&t<=5);
VZ=ZV_2.*(t>=0&t<3)+ZV_1.*(t>=3&t<=5);
aZ=Za_2.*(t>=0&t<3)+Za_1.*(t>=3&t<=5);

dpt=[X,Y,Z];V=[VX,VY,VZ]; a=[aX,aY,aZ].';


else
    

[K_1,KV_1,Ka_1]=polynomial_v(t,2, 550, 0,0, 450,-90,-30);%4-6
[K_2,KV_2,Ka_2]=polynomial_v((t-2),1, 450,-90,-30, 350,-120,-10);%6-7
[K_3,KV_3,Ka_3]=polynomial_v((t-3),1, 350,-120,-10, 250,-100,-10);%7-8
[K_4,KV_4,Ka_4]=polynomial_v((t-4),2, 250,-100,-10,150,0,0);%8-10
K_5=150;KV_5=0;Ka_5=0;
X=K_1.*(t>=0&t<2)+K_2.*(t>=2&t<3)+K_3.*(t>=3&t<4)+K_4.*(t>=4&t<6)+K_5.*(t>=6&t<=10);
VX=KV_1.*(t>=0&t<2)+KV_2.*(t>=2&t<3)+KV_3.*(t>=3&t<4)+KV_4.*(t>=4&t<6)+KV_5.*(t>=6&t<=10);
aX=Ka_1.*(t>=0&t<2)+Ka_2.*(t>=2&t<3)+Ka_3.*(t>=3&t<4)+Ka_4.*(t>=4&t<6)+Ka_5.*(t>=6&t<=10);



[S_1,SV_1,Sa_1]=polynomial_v(t,2, 225,0,0, 180,-40,20);%4-6s
[S_2,SV_2,Sa_2]=polynomial_v((t-2),1, 180,-40,20, 150,-50,40);%6-7s
[S_3,SV_3,Sa_3]=polynomial_v((t-3),1, 150,-50,40, 100,-10,10);%7-8s
[S_4,SV_4,Sa_4]=polynomial_v((t-4),2, 100,-10,10, 0,0,0);%8-10s
S_5=0;SV_5=0;Sa_5=0;
Y=S_1.*(t>=0&t<2)+S_2.*(t>=2&t<3)+S_3.*(t>=3&t<4)+S_4.*(t>=4&t<6)+S_5.*(t>=6&t<=10);
VY=SV_1.*(t>=0&t<2)+SV_2.*(t>=2&t<3)+SV_3.*(t>=3&t<4)+SV_4.*(t>=4&t<6)+SV_5.*(t>=6&t<=10);
aY=Sa_1.*(t>=0&t<2)+Sa_2.*(t>=2&t<3)+Sa_3.*(t>=3&t<4)+Sa_4.*(t>=4&t<6)+Sa_5.*(t>=6&t<=10);

[Z_1,ZV_1,Za_1]=polynomial_v((t-6),4,980,0,0,1300,0,0);
Z_2=980;ZV_2=0;Za_2=0;
Z=Z_2.*(t>=0&t<6)+Z_1.*(t>=6&t<=10);
VZ=ZV_2.*(t>=0&t<6)+ZV_1.*(t>=6&t<=10);
aZ=Za_2.*(t>=0&t<6)+Za_1.*(t>=6&t<=10);

dpt=[X,Y,Z];V=[VX,VY,VZ]; a=[aX,aY,aZ].';

end
end

== matlab function new_inkine_2020/MATLAB Function3 ==
  data: t input; dpt output; V output; a output; flag input
function [dpt,V,a] = TRACE_NEW1(t,flag)%轨迹规划
if flag==1
K_1=0;KV_1=0;Ka_1=0;
[K_2,KV_2,Ka_2]=polynomial_v((t-2),1, 0,0,0, 125,180,10);%2-3
[K_3,KV_3,Ka_3]=polynomial_v((t-3),0.5, 125,180,10, 225,200,-60);%3-3.5
[K_4,KV_4,Ka_4]=polynomial_v((t-3.5),0.5, 225,200,-60, 325,200,120);%3.5-4
[K_5,KV_5,Ka_5]=polynomial_v((t-4),1, 325,200,120, 475, 0,0);%4-5
X=K_1.*(t>=0&t<2)+K_2.*(t>=2&t<3)+K_3.*(t>=3&t<3.5)+K_4.*(t>=3.5&t<4)+K_5.*(t>=4&t<=5);
VX=KV_1.*(t>=0&t<2)+KV_2.*(t>=2&t<3)+KV_3.*(t>=3&t<3.5)+KV_4.*(t>=3.5&t<4)+KV_5.*(t>=4&t<=5);
aX=Ka_1.*(t>=0&t<2)+Ka_2.*(t>=2&t<3)+Ka_3.*(t>=3&t<3.5)+Ka_4.*(t>=3.5&t<4)+Ka_5.*(t>=4&t<=5);

S_1=225;SV_1=0;Sa_1=0;
[S_2,SV_2,Sa_2]=polynomial_v((t-2),1, 225,0,0, 90,-120,210);%2-3s
[S_3,SV_3,Sa_3]=polynomial_v((t-3),0.5, 90,-120,210, 45,-75,45);%3-3.5s
[S_4,SV_4,Sa_4]=polynomial_v((t-3.5),0.5, 45,-75,45, 20,-36,10);%3.5-4s
[S_5,SV_5,Sa_5]=polynomial_v((t-4),1, 20,-36,10, 0, 0,0);%4-5s
Y=S_1.*(t>=0&t<2)+S_2.*(t>=2&t<3)+S_3.*(t>=3&t<3.5)+S_4.*(t>=3.5&t<4)+S_5.*(t>=4&t<=5);
VY=SV_1.*(t>=0&t<2)+SV_2.*(t>=2&t<3)+SV_3.*(t>=3&t<3.5)+SV_4.*(t>=3.5&t<4)+SV_5.*(t>=4&t<=5);
aY=Sa_1.*(t>=0&t<2)+Sa_2.*(t>=2&t<3)+Sa_3.*(t>=3&t<3.5)+Sa_4.*(t>=3.5&t<4)+Sa_5.*(t>=4&t<=5);

[Z_1,ZV_1,Za_1]=polynomial_v(t,2,1300,0,0,1000,0,0);
Z_2=1000;ZV_2=0;Za_2=0;
Z=Z_1.*(t>=0&t<2)+Z_2.*(t>=2&t<=5);
VZ=ZV_1.*(t>=0&t<2)+ZV_2.*(t>=2&t<=5);
aZ=Za_1.*(t>=0&t<2)+Za_2.*(t>=2&t<=5);

dpt=[X,Y,Z];V=[VX,VY,VZ]; a=[aX,aY,aZ].';


elseif flag==2
    
K_1=0;KV_1=0;Ka_1=0;
[K_2,KV_2,Ka_2]=polynomial_v((t-4),2, 0,0,0, 125,90,10);%4-6
[K_3,KV_3,Ka_3]=polynomial_v((t-6),1, 125,90,10, 225,100,0);%6-7
[K_4,KV_4,Ka_4]=polynomial_v((t-7),1, 225,100,0, 325,100,20);%7-8
[K_5,KV_5,Ka_5]=polynomial_v((t-8),2, 325,100,20, 475, 0,0);%8-10
X=K_1.*(t>=0&t<4)+K_2.*(t>=4&t<6)+K_3.*(t>=6&t<7)+K_4.*(t>=7&t<8)+K_5.*(t>=8&t<=10);
VX=KV_1.*(t>=0&t<4)+KV_2.*(t>=4&t<6)+KV_3.*(t>=6&t<7)+KV_4.*(t>=7&t<8)+KV_5.*(t>=8&t<=10);
aX=Ka_1.*(t>=0&t<4)+Ka_2.*(t>=4&t<6)+Ka_3.*(t>=6&t<7)+Ka_4.*(t>=7&t<8)+Ka_5.*(t>=8&t<=10);


S_1=225;SV_1=0;Sa_1=0;
[S_2,SV_2,Sa_2]=polynomial_v((t-4),2, 225,0,0, 90,-60,60);%4-6s
[S_3,SV_3,Sa_3]=polynomial_v((t-6),1, 90,-60,60, 45,-35,20);%6-7s
[S_4,SV_4,Sa_4]=polynomial_v((t-7),1, 45,-35,20, 20,-18,10);%7-8s
[S_5,SV_5,Sa_5]=polynomial_v((t-8),2, 20,-18,10, 0, 0,0);%8-10s
Y=S_1.*(t>=0&t<4)+S_2.*(t>=4&t<6)+S_3.*(t>=6&t<7)+S_4.*(t>=7&t<8)+S_5.*(t>=8&t<=10);
VY=SV_1.*(t>=0&t<4)+SV_2.*(t>=4&t<6)+SV_3.*(t>=6&t<7)+SV_4.*(t>=7&t<8)+SV_5.*(t>=8&t<=10);
aY=Sa_1.*(t>=0&t<4)+Sa_2.*(t>=4&t<6)+Sa_3.*(t>=6&t<7)+Sa_4.*(t>=7&t<8)+Sa_5.*(t>=8&t<=10);

[Z_1,ZV_1,Za_1]=polynomial_v(t,4,1300,0,0,1000,0,0);
Z_2=1000;ZV_2=0;Za_2=0;
Z=Z_1.*(t>=0&t<4)+Z_2.*(t>=4&t<=10);
VZ=ZV_1.*(t>=0&t<4)+ZV_2.*(t>=4&t<=10);
aZ=Za_1.*(t>=0&t<4)+Za_2.*(t>=4&t<=10);

dpt=[X,Y,Z];V=[VX,VY,VZ]; a=[aX,aY,aZ].';

else
K_1=150;KV_1=0;Ka_1=0;
[K_2,KV_2,Ka_2]=polynomial_v((t-6),3, 150,0,0, 250,60,5);%6-9
[K_3,KV_3,Ka_3]=polynomial_v((t-9),1.5, 250,60,5, 350,65,0);%9-10.5
[K_4,KV_4,Ka_4]=polynomial_v((t-10.5),1.5, 350,65,0, 450,65,7);%10.5-12
[K_5,KV_5,Ka_5]=polynomial_v((t-12),3, 450,65,7, 550, 0,0);%12-15
X=K_1.*(t>=0&t<6)+K_2.*(t>=6&t<9)+K_3.*(t>=9&t<10.5)+K_4.*(t>=10.5&t<12)+K_5.*(t>=12&t<=15);
VX=KV_1.*(t>=0&t<6)+KV_2.*(t>=6&t<9)+KV_3.*(t>=9&t<10.5)+KV_4.*(t>=10.5&t<12)+KV_5.*(t>=12&t<=15);
aX=Ka_1.*(t>=0&t<6)+Ka_2.*(t>=6&t<9)+Ka_3.*(t>=9&t<10.5)+Ka_4.*(t>=10.5&t<12)+Ka_5.*(t>=12&t<=15);


S_1=0;SV_1=0;Sa_1=0;
[S_2,SV_2,Sa_2]=polynomial_v((t-6),3, 0,0,0, 100,40,20);%4-6s
[S_3,SV_3,Sa_3]=polynomial_v((t-9),1.5, 100,40,20, 150,24,5);%6-7s
[S_4,SV_4,Sa_4]=polynomial_v((t-10.5),1.5, 150,24,5, 180,12,5);%7-8s
[S_5,SV_5,Sa_5]=polynomial_v((t-12),3, 180,12,5, 225, 0,0);%8-10s
Y=S_1.*(t>=0&t<6)+S_2.*(t>=6&t<9)+S_3.*(t>=9&t<10.5)+S_4.*(t>=10.5&t<12)+S_5.*(t>=12&t<=15);
VY=SV_1.*(t>=0&t<6)+SV_2.*(t>=6&t<9)+SV_3.*(t>=9&t<10.5)+SV_4.*(t>=10.5&t<12)+SV_5.*(t>=12&t<=15);
aY=Sa_1.*(t>=0&t<6)+Sa_2.*(t>=6&t<9)+Sa_3.*(t>=9&t<10.5)+Sa_4.*(t>=10.5&t<12)+Sa_5.*(t>=12&t<=15);

[Z_1,ZV_1,Za_1]=polynomial_v(t,6,1300,0,0,1000,0,0);
Z_2=1000;ZV_2=0;Za_2=0;
Z=Z_1.*(t>=0&t<6)+Z_2.*(t>=6&t<=15);
VZ=ZV_1.*(t>=0&t<6)+ZV_2.*(t>=6&t<=15);
aZ=Za_1.*(t>=0&t<6)+Za_2.*(t>=6&t<=15);

dpt=[X,Y,Z];V=[VX,VY,VZ]; a=[aX,aY,aZ].';
end
end

== matlab function new_inkine_2020/MATLAB Function5 ==
  data: t input; dpt output; V output; a output; flag input
function [dpt,V,a] = TRACE_1A(t,flag)%轨迹规划
    if flag==0
        [K_1, KV_1, Ka_1] = polynomial_v(t, 2, 0, 0, 0, 150, 100, 0); % 4-6
        [K_2, KV_2, Ka_2] = polynomial_v((t-2), 1, 150, 100, 0, 250, 100, 0); % 6-7
        [K_3, KV_3, Ka_3] = polynomial_v((t-3), 1, 250, 100, 0, 350, 100, 0); % 7-8
        [K_4, KV_4, Ka_4] = polynomial_v((t-4), 2, 350, 100, 0, 500, 0, 0); % 8-10
        K_5 = 500; KV_5 = 0; Ka_5 = 0;
        X = K_1.*(t>=0 & t<2) + K_2.*(t>=2 & t<3) + K_3.*(t>=3 & t<4) + K_4.*(t>=4 & t<6) + K_5.*(t>=6 & t<=10);
        VX = KV_1.*(t>=0 & t<2) + KV_2.*(t>=2 & t<3) + KV_3.*(t>=3 & t<4) + KV_4.*(t>=4 & t<6) + KV_5.*(t>=6 & t<=10);
        aX = Ka_1.*(t>=0 & t<2) + Ka_2.*(t>=2 & t<3) + Ka_3.*(t>=3 & t<4) + Ka_4.*(t>=4 & t<6) + Ka_5.*(t>=6 & t<=10);

        [S_1, SV_1, Sa_1] = polynomial_v(t, 2, 500, 0, 0, 420, -96, -12); % 4-6s
        [S_2, SV_2, Sa_2] = polynomial_v((t-2), 1, 420, -96, -12, 330, -82, 17); % 6-7s
        [S_3, SV_3, Sa_3] = polynomial_v((t-3), 1, 330, -82, 17, 255, -69, 23); % 7-8s
        [S_4, SV_4, Sa_4] = polynomial_v((t-4), 2, 255, -69, 23, 200, 0, 0); % 8-10s
        S_5 = 200; SV_5 = 0; Sa_5 = 0;
        Y = S_1.*(t>=0 & t<2) + S_2.*(t>=2 & t<3) + S_3.*(t>=3 & t<4) + S_4.*(t>=4 & t<6) + S_5.*(t>=6 & t<=10);
        VY = SV_1.*(t>=0 & t<2) + SV_2.*(t>=2 & t<3) + SV_3.*(t>=3 & t<4) + SV_4.*(t>=4 & t<6) + SV_5.*(t>=6 & t<=10);
        aY = Sa_1.*(t>=0 & t<2) + Sa_2.*(t>=2 & t<3) + Sa_3.*(t>=3 & t<4) + Sa_4.*(t>=4 & t<6) + Sa_5.*(t>=6 & t<=10);

        [Z_1, ZV_1, Za_1] = polynomial_v((t-6), 4, 950, 0, 0, 1202, 0, 0);
        Z_2 = 950; ZV_2 = 0; Za_2 = 0;
        Z = Z_2.*(t>=0 & t<6) + Z_1.*(t>=6 & t<=10);
        VZ = ZV_2.*(t>=0 & t<6) + ZV_1.*(t>=6 & t<=10);
        aZ = Za_2.*(t>=0 & t<6) + Za_1.*(t>=6 & t<=10);

        dpt=[X,Y,Z];V=[VX,VY,VZ]; a=[aX,aY,aZ].';
        
%     elseif flag==1
    else
        [K_1, KV_1, Ka_1] = polynomial_v(t, 2, 0, 0, 0, -150, -100, 0); % 4-6
        [K_2, KV_2, Ka_2] = polynomial_v((t-2), 1, -150, -100, 0, -250, -100, 0); % 6-7
        [K_3, KV_3, Ka_3] = polynomial_v((t-3), 1, -250, -100, 0, -350, -100, 0); % 7-8
        [K_4, KV_4, Ka_4] = polynomial_v((t-4), 2, -350, -100, 0, -500, 0, 0); % 8-10
        K_5 = -500; KV_5 = 0; Ka_5 = 0;
        X = K_1.*(t>=0 & t<2) + K_2.*(t>=2 & t<3) + K_3.*(t>=3 & t<4) + K_4.*(t>=4 & t<6) + K_5.*(t>=6 & t<=10);
        VX = KV_1.*(t>=0 & t<2) + KV_2.*(t>=2 & t<3) + KV_3.*(t>=3 & t<4) + KV_4.*(t>=4 & t<6) + KV_5.*(t>=6 & t<=10);
        aX = Ka_1.*(t>=0 & t<2) + Ka_2.*(t>=2 & t<3) + Ka_3.*(t>=3 & t<4) + Ka_4.*(t>=4 & t<6) + Ka_5.*(t>=6 & t<=10);

        [S_1, SV_1, Sa_1] = polynomial_v(t, 2, 500, 0, 0, 420, -96, -12); % 4-6s
        [S_2, SV_2, Sa_2] = polynomial_v((t-2), 1, 420, -96, -12, 330, -82, 17); % 6-7s
        [S_3, SV_3, Sa_3] = polynomial_v((t-3), 1, 330, -82, 17, 255, -69, 23); % 7-8s
        [S_4, SV_4, Sa_4] = polynomial_v((t-4), 2, 255, -69, 23, 200, 0, 0); % 8-10s
        S_5 = 200; SV_5 = 0; Sa_5 = 0;
        Y = S_1.*(t>=0 & t<2) + S_2.*(t>=2 & t<3) + S_3.*(t>=3 & t<4) + S_4.*(t>=4 & t<6) + S_5.*(t>=6 & t<=10);
        VY = SV_1.*(t>=0 & t<2) + SV_2.*(t>=2 & t<3) + SV_3.*(t>=3 & t<4) + SV_4.*(t>=4 & t<6) + SV_5.*(t>=6 & t<=10);
        aY = Sa_1.*(t>=0 & t<2) + Sa_2.*(t>=2 & t<3) + Sa_3.*(t>=3 & t<4) + Sa_4.*(t>=4 & t<6) + Sa_5.*(t>=6 & t<=10);

        [Z_1, ZV_1, Za_1] = polynomial_v((t-6), 4, 950, 0, 0, 1200, 0, 0);
        Z_2 = 950; ZV_2 = 0; Za_2 = 0;
        Z = Z_2.*(t>=0 & t<6) + Z_1.*(t>=6 & t<=10);
        VZ = ZV_2.*(t>=0 & t<6) + ZV_1.*(t>=6 & t<=10);
        aZ = Za_2.*(t>=0 & t<6) + Za_1.*(t>=6 & t<=10);

        dpt=[X,Y,Z];V=[VX,VY,VZ]; a=[aX,aY,aZ].';

    end
end

== matlab function new_inkine_2020/MATLAB Function8 ==
  data: t input; dpt output; V output; a output; flag input
function [dpt,V,a] = TRACE_1B(t,flag)%轨迹规划
if flag==0
K_1=500;KV_1=0;Ka_1=0;
[K_2,KV_2,Ka_2]=polynomial_v((t-4),2, 500,0,0, 350,-100,0);%4-6
[K_3,KV_3,Ka_3]=polynomial_v((t-6),1, 350,-100,0, 250,-100,0);%6-7
[K_4,KV_4,Ka_4]=polynomial_v((t-7),1, 250,-100,0, 150,-100,0);%7-8
[K_5,KV_5,Ka_5]=polynomial_v((t-8),2, 150,-100,0, 0, 0,0);%8-10
X=K_1.*(t>=0&t<4)+K_2.*(t>=4&t<6)+K_3.*(t>=6&t<7)+K_4.*(t>=7&t<8)+K_5.*(t>=8&t<=10);
VX=KV_1.*(t>=0&t<4)+KV_2.*(t>=4&t<6)+KV_3.*(t>=6&t<7)+KV_4.*(t>=7&t<8)+KV_5.*(t>=8&t<=10);
aX=Ka_1.*(t>=0&t<4)+Ka_2.*(t>=4&t<6)+Ka_3.*(t>=6&t<7)+Ka_4.*(t>=7&t<8)+Ka_5.*(t>=8&t<=10);


S_1=200;SV_1=0;Sa_1=0;
[S_2,SV_2,Sa_2]=polynomial_v((t-4),2, 200,0,0, 255,69,23);%4-6s
[S_3,SV_3,Sa_3]=polynomial_v((t-6),1, 255,69,23, 330,82,17);%6-7s
[S_4,SV_4,Sa_4]=polynomial_v((t-7),1, 330,82,17, 420,96,-12);%7-8s
[S_5,SV_5,Sa_5]=polynomial_v((t-8),2, 420,96,-12, 500, 0,0);%8-10s
Y=S_1.*(t>=0&t<4)+S_2.*(t>=4&t<6)+S_3.*(t>=6&t<7)+S_4.*(t>=7&t<8)+S_5.*(t>=8&t<=10);
VY=SV_1.*(t>=0&t<4)+SV_2.*(t>=4&t<6)+SV_3.*(t>=6&t<7)+SV_4.*(t>=7&t<8)+SV_5.*(t>=8&t<=10);
aY=Sa_1.*(t>=0&t<4)+Sa_2.*(t>=4&t<6)+Sa_3.*(t>=6&t<7)+Sa_4.*(t>=7&t<8)+Sa_5.*(t>=8&t<=10);

[Z_1,ZV_1,Za_1]=polynomial_v(t,4,1200,0,0,950,0,0);
Z_2=950;ZV_2=0;Za_2=0;
Z=Z_1.*(t>=0&t<4)+Z_2.*(t>=4&t<=10);
VZ=ZV_1.*(t>=0&t<4)+ZV_2.*(t>=4&t<=10);
aZ=Za_1.*(t>=0&t<4)+Za_2.*(t>=4&t<=10);

dpt=[X,Y,Z];V=[VX,VY,VZ]; a=[aX,aY,aZ].';

else
K_1=-500;KV_1=0;Ka_1=0;
[K_2,KV_2,Ka_2]=polynomial_v((t-4),2, -500,0,0, -350,100,0);%4-6
[K_3,KV_3,Ka_3]=polynomial_v((t-6),1, -350,100,0, -250,100,0);%6-7
[K_4,KV_4,Ka_4]=polynomial_v((t-7),1, -250,100,0, -150,100,0);%7-8
[K_5,KV_5,Ka_5]=polynomial_v((t-8),2, -150,100,-0, 0, 0,0);%8-10
X=K_1.*(t>=0&t<4)+K_2.*(t>=4&t<6)+K_3.*(t>=6&t<7)+K_4.*(t>=7&t<8)+K_5.*(t>=8&t<=10);
VX=KV_1.*(t>=0&t<4)+KV_2.*(t>=4&t<6)+KV_3.*(t>=6&t<7)+KV_4.*(t>=7&t<8)+KV_5.*(t>=8&t<=10);
aX=Ka_1.*(t>=0&t<4)+Ka_2.*(t>=4&t<6)+Ka_3.*(t>=6&t<7)+Ka_4.*(t>=7&t<8)+Ka_5.*(t>=8&t<=10);

S_1=200;SV_1=0;Sa_1=0;
[S_2,SV_2,Sa_2]=polynomial_v((t-4),2, 200,0,0, 255,69,23);%4-6s
[S_3,SV_3,Sa_3]=polynomial_v((t-6),1, 255,69,23, 330,82,17);%6-7s
[S_4,SV_4,Sa_4]=polynomial_v((t-7),1, 330,82,17, 420,96,-12);%7-8s
[S_5,SV_5,Sa_5]=polynomial_v((t-8),2, 420,96,-12, 500, 0,0);%8-10s
Y=S_1.*(t>=0&t<4)+S_2.*(t>=4&t<6)+S_3.*(t>=6&t<7)+S_4.*(t>=7&t<8)+S_5.*(t>=8&t<=10);
VY=SV_1.*(t>=0&t<4)+SV_2.*(t>=4&t<6)+SV_3.*(t>=6&t<7)+SV_4.*(t>=7&t<8)+SV_5.*(t>=8&t<=10);
aY=Sa_1.*(t>=0&t<4)+Sa_2.*(t>=4&t<6)+Sa_3.*(t>=6&t<7)+Sa_4.*(t>=7&t<8)+Sa_5.*(t>=8&t<=10);

[Z_1,ZV_1,Za_1]=polynomial_v(t,4,1200,0,0,950,0,0);
Z_2=950;ZV_2=0;Za_2=0;
Z=Z_1.*(t>=0&t<4)+Z_2.*(t>=4&t<=10);
VZ=ZV_1.*(t>=0&t<4)+ZV_2.*(t>=4&t<=10);
aZ=Za_1.*(t>=0&t<4)+Za_2.*(t>=4&t<=10);

dpt=[X,Y,Z];V=[VX,VY,VZ]; a=[aX,aY,aZ].';
end
end

== matlab function new_inkine_2020/MATLAB Function9 ==
  data: t input; dpt output; V output; a output; flag input
function [dpt,V,a] = TRACE_1C(t,flag)%轨迹规划
    if flag==0
        P1xyz=[100, 200, 950];
        P2xyz=[0, 500, 950];
        P3xyz=[-80, 200, 950];
%         N1=4998; N2=4999; % 插值点的个数
        T_total=10;
%         t=linspace(0,10,10000);
        [P,V]= traj_plan_circle(P1xyz, P2xyz, P3xyz,T_total,t);
        X=P(:,1);
        Y=P(:,2);
        Z=P(:,3);
        % 计算速度和加速度
        V_X=V(:,1);
        V_Y=V(:,2);
        V_Z=V(:,3);   
%         a_X=a(:,1);
%         a_Y=a(:,2);
%         a_Z=a(:,3);
        dpt=[X,Y,Z];
        V=[V_X,V_Y,V_Z];
        a=[X,Y,Z].';
%         V=[V_X,V_Y,V_Z];
%         a=[a_X,a_Y,a_Z];
    else
        P1xyz=[100, 200, 950];
        P2xyz=[0, 500, 950];
        P3xyz=[-100, 200, 950];
%         N1=4998; N2=4999; % 插值点的个数
        T_total=10;
%         t=linspace(0,10,10000);
        [P]= traj_plan_circle(P1xyz, P2xyz, P3xyz,T_total,t);
        X=P(:,1);
        Y=P(:,2);
        Z=P(:,3);
        % 计算速度和加速度
%         V_X=V(:,1);
%         V_Y=V(:,2);
%         V_Z=V(:,3);   
%         a_X=a(:,1);
%         a_Y=a(:,2);
%         a_Z=a(:,3);
        dpt=[X,Y,Z];
        V=[X,Y,Z];
        a=[X,Y,Z].';
%         V=[V_X,V_Y,V_Z];
%         a=[a_X,a_Y,a_Z];
        

    end
end

== matlab function new_inkine_2020/MATLAB Function10 ==
  data: t input; dpt output; V output; a output; flag input
% function [dpt,V,a] = TRACE_Access(t,flag)%轨迹规划
% if flag==1
% [K_1,KV_1,Ka_1]=polynomial_v(t,1, 475, 0,0, 325,-200,60);%0-1
% [K_2,KV_2,Ka_2]=polynomial_v((t-1),0.5, 325,-200,60, 225,-200,-20);%1-1.5
% [K_3,KV_3,Ka_3]=polynomial_v((t-1.5),0.5, 225,-200,-20, 125,-180,-0);%1.5-2
% [K_4,KV_4,Ka_4]=polynomial_v((t-2),1, 125,-180,-10, 0,0,0);%2-3
% K_5=0;KV_5=0;Ka_5=0;
% X=K_1.*(t>=0&t<1)+K_2.*(t>=1&t<1.5)+K_3.*(t>=1.5&t<2)+K_4.*(t>=2&t<3)+K_5.*(t>=3&t<=5);
% VX=KV_1.*(t>=0&t<1)+KV_2.*(t>=1&t<1.5)+KV_3.*(t>=1.5&t<2)+KV_4.*(t>=2&t<3)+KV_5.*(t>=3&t<=5);
% aX=Ka_1.*(t>=0&t<1)+Ka_2.*(t>=1&t<1.5)+Ka_3.*(t>=1.5&t<2)+Ka_4.*(t>=2&t<3)+Ka_5.*(t>=3&t<=5);
% 
% [S_1,SV_1,Sa_1]=polynomial_v(t,1, 0,0,0, 20,36,-10);%0-1s
% [S_2,SV_2,Sa_2]=polynomial_v((t-1),0.5, 20,36,-10, 45,75,25);%1-1.5s
% [S_3,SV_3,Sa_3]=polynomial_v((t-1.5),0.5, 45,75,25, 90,150,300);%1.5-2s
% [S_4,SV_4,Sa_4]=polynomial_v((t-2),1, 90,150,300, 225,0,0);%2-3s
% S_5=225;SV_5=0;Sa_5=0;
% 
% Y=S_1.*(t>=0&t<1)+S_2.*(t>=1&t<1.5)+S_3.*(t>=1.5&t<2)+S_4.*(t>=2&t<3)+S_5.*(t>=3&t<=5);
% VY=SV_1.*(t>=0&t<1)+SV_2.*(t>=1&t<1.5)+SV_3.*(t>=1.5&t<2)+SV_4.*(t>=2&t<3)+SV_5.*(t>=3&t<=5);
% aY=Sa_1.*(t>=0&t<1)+Sa_2.*(t>=1&t<1.5)+Sa_3.*(t>=1.5&t<2)+Sa_4.*(t>=2&t<3)+Sa_5.*(t>=3&t<=5);
% 
% [Z_1,ZV_1,Za_1]=polynomial_v((t-3),2,980,0,0,1300,0,0);
% Z_2=980;ZV_2=0;Za_2=0;
% Z=Z_2.*(t>=0&t<3)+Z_1.*(t>=3&t<=5);
% VZ=ZV_2.*(t>=0&t<3)+ZV_1.*(t>=3&t<=5);
% aZ=Za_2.*(t>=0&t<3)+Za_1.*(t>=3&t<=5);
% 
% dpt=[X,Y,Z];V=[VX,VY,VZ]; a=[aX,aY,aZ].';
% 
% 
% else
%     
% 
% [K_1,KV_1,Ka_1]=polynomial_v(t,2, 475, 0,0, 325,-90,20);%4-6
% [K_2,KV_2,Ka_2]=polynomial_v((t-2),1, 325,-90,20, 225,-120,-10);%6-7
% [K_3,KV_3,Ka_3]=polynomial_v((t-3),1, 225,-120,-10, 125,-100,-20);%7-8
% [K_4,KV_4,Ka_4]=polynomial_v((t-4),2, 125,-100,-20 , 0,0,0);%8-10
% K_5=0;KV_5=0;Ka_5=0;
% X=K_1.*(t>=0&t<2)+K_2.*(t>=2&t<3)+K_3.*(t>=3&t<4)+K_4.*(t>=4&t<6)+K_5.*(t>=6&t<=10);
% VX=KV_1.*(t>=0&t<2)+KV_2.*(t>=2&t<3)+KV_3.*(t>=3&t<4)+KV_4.*(t>=4&t<6)+KV_5.*(t>=6&t<=10);
% aX=Ka_1.*(t>=0&t<2)+Ka_2.*(t>=2&t<3)+Ka_3.*(t>=3&t<4)+Ka_4.*(t>=4&t<6)+Ka_5.*(t>=6&t<=10);
% 
% 
% 
% [S_1,SV_1,Sa_1]=polynomial_v(t,2, 0,0,0, 20,15,15);%4-6s
% [S_2,SV_2,Sa_2]=polynomial_v((t-2),1, 20,15,15, 45,30,-10);%6-7s
% [S_3,SV_3,Sa_3]=polynomial_v((t-3),1, 45,30,-10, 90,80,80);%7-8s
% [S_4,SV_4,Sa_4]=polynomial_v((t-4),2, 90,80,80, 225,0,0);%8-10s
% S_5=225;SV_5=0;Sa_5=0;
% Y=S_1.*(t>=0&t<2)+S_2.*(t>=2&t<3)+S_3.*(t>=3&t<4)+S_4.*(t>=4&t<6)+S_5.*(t>=6&t<=10);
% VY=SV_1.*(t>=0&t<2)+SV_2.*(t>=2&t<3)+SV_3.*(t>=3&t<4)+SV_4.*(t>=4&t<6)+SV_5.*(t>=6&t<=10);
% aY=Sa_1.*(t>=0&t<2)+Sa_2.*(t>=2&t<3)+Sa_3.*(t>=3&t<4)+Sa_4.*(t>=4&t<6)+Sa_5.*(t>=6&t<=10);
% 
% [Z_1,ZV_1,Za_1]=polynomial_v((t-6),4,980,0,0,1300,0,0);
% Z_2=980;ZV_2=0;Za_2=0;
% Z=Z_2.*(t>=0&t<6)+Z_1.*(t>=6&t<=10);
% VZ=ZV_2.*(t>=0&t<6)+ZV_1.*(t>=6&t<=10);
% aZ=Za_2.*(t>=0&t<6)+Za_1.*(t>=6&t<=10);
% 
% dpt=[X,Y,Z];V=[VX,VY,VZ]; a=[aX,aY,aZ].';
% 
% 
% % end
% % end
% function [dpt,V,a] = TRACE_Access(t,flag)
%     % 直线轨迹参数（以flag==1为例）
%     start_point = [0, 0, 980];   % 起点[X,Y,Z]
%     end_point = [100, 200, 1300];% 终点
%     linear_duration = 2;         % 持续时间2秒
%     linear_start = 3;            % 第3秒开始

%     if flag == 1
%         % X轴直线分量
%         if t >= linear_start && t <= (linear_start + linear_duration)
%             [X, VX, aX] = linear_interp(t-linear_start, linear_duration,...
%                 start_point(1), end_point(1));
%         else
%             X = 0; VX = 0; aX = 0; % 其他时间段归零
%         end
%         
%         % Y轴直线分量（同上逻辑）
%         if t >= linear_start && t <= (linear_start + linear_duration)
%             [Y, VY, aY] = linear_interp(t-linear_start, linear_duration,...
%                 start_point(2), end_point(2));
%         else
%             Y = 0; VY = 0; aY = 0;
%         end
%         
%         % Z轴直线分量 
%         if t >= linear_start && t <= (linear_start + linear_duration)
%             [Z, VZ, aZ] = linear_interp(t-linear_start, linear_duration,...
%                 start_point(3), end_point(3));
%         else
%             Z = 980; VZ = 0; aZ = 0; % 保持初始高度
%         end
%         
%         dpt = [X, Y, Z];
%         V = [VX, VY, VZ];
%         a = [aX, aY, aZ].';
%     else
%         % flag==0的其他模式（保持原有逻辑）
%     end 
% end






% %直线插补
% function [dpt,V,a] = TRACE_Access(t,flag)%轨迹规划
%  if flag==1
%   [X,XV,Xa]=linear_interp(t, 10,475, 0);
%   [Y,YV,Ya]=linear_interp(t, 10,0, 225);
%   [Z,ZV,Za]=linear_interp(t,10,980,1000);
%   dpt=[X,Y,Z];V=[XV,YV,ZV]; a=[Xa,Ya,Za];
%   else


% function [dpt,V,a] = TRACE_Access(t,flag)%轨迹规划
%  if flag==1
%  %x轴
%      [K_1,KV_1,Ka_1]=polynomial_v(t,2, 475, 0,0, 425,37.5,0);%0-2加速  
%      [K_2,KV_2,Ka_2]=linear_interp((t-2), 10,425, 50);%2-12匀速速
%      [K_3,KV_3,Ka_3]=polynomial_v((t-12),2, 50,37.5,0, 0,0,0);%12-14减速
%      X=K_1.*(t>=0&t<2)+K_2.*(t>=2&t<12)+K_3.*(t>=12&t<14);
%      VX=KV_1.*(t>=0&t<2)+KV_2.*(t>=2&t<3)+KV_3.*(t>=3&t<4);
%      aX=Ka_1.*(t>=0&t<2)+Ka_2.*(t>=2&t<3)+Ka_3.*(t>=3&t<4);
%  %y轴    
%      [S_1,SV_1,Sa_1]=polynomial_v(t,2, 0,0,0, 50,12.5,0);%4-6s
%      [S_2,SV_2,Sa_2]=linear_interp((t-2), 10,50, 175);
%      [S_3,SV_3,Sa_3]=polynomial_v((t-12),2, 175,12.5,0, 225,0,0);%7-8s
%      Y=S_1.*(t>=0&t<2)+S_2.*(t>=2&t<12)+S_3.*(t>=12&t<14);
%      VY=SV_1.*(t>=0&t<2)+SV_2.*(t>=2&t<12)+SV_3.*(t>=12&t<14);
%      aY=Sa_1.*(t>=0&t<2)+Sa_2.*(t>=2&t<12)+Sa_3.*(t>=12&t<14);
%  %z轴
%      [Z_1,ZV_1,Za_1]=polynomial_v(t,2,980,0,0,1030,22,0);
%      [Z_2,ZV_2,Za_2]=linear_interp((t-2),10,1030,1250);
%      [Z_3,ZV_3,Za_3]=polynomial_v((t-12),2,1250,22,0,1300,0,0);
%      Z=Z_2.*(t>=0&t<2)+Z_1.*(t>=2&t<=12)+Z_3.*(t>=12&t<=14);
%      VZ=ZV_2.*(t>=0&t<2)+ZV_1.*(t>=2&t<=12)+ZV_3.*(t>=12&t<=14);
%      aZ=Za_2.*(t>=0&t<2)+Za_1.*(t>=2&t<=12)+Za_3.*(t>=12&t<=14);
%  
%      dpt=[X,Y,Z];V=[VX,VY,VZ]; a=[aX,aY,aZ];
%   else





% function [dpt,V,a] = TRACE_Access(t,flag)%轨迹规划
% 
% if flag==1
%   % 参数设置
% s_start = [475, 0, 980];  % 初始位置 [x_start, y_start, z_start]
% s_end = [0, 225, 1300];   % 终止位置 [x_end, y_end, z_end]
% v_max = 150;            % 最大速度 (m/s)
% a_max = 50;            % 最大加速度 (m/s²)
% t = 7.1;         % 总时间 (s)
% % 初始化输出
%     dpt = zeros(3, 1000);
%     V = zeros(3, 1000);
%     a = zeros(3, 1000);
% 
%     % 对每个自由度进行计算
%     for dim = 1:3
%         % 调用之前定义的函数
%         [position, velocity, acceleration] = trapezoidal_velocity_profile(t,s_start(dim), s_end(dim), v_max(dim), a_max(dim));
%      
%         % 将结果存储到输出矩阵中
%         dpt(dim, :) = position;
%         V(dim, :) = velocity;
%         a(dim, :) = acceleration;
%     end

% % 轨迹规划
% [position_x, velocity_x, acceleration_x] = trapezoidal_velocity_profile(t_total, s_start(1), s_end(1), v_max, a_max);
% [position_y, velocity_y, acceleration_y] = trapezoidal_velocity_profile(t_total, s_start(2), s_end(2), v_max, a_max);
% [position_z, velocity_z, acceleration_z] = trapezoidal_velocity_profile(t_total, s_start(3), s_end(3), v_max, a_max);
% 
% % 合并输出
% dpt = [position_x(:); position_y(:); position_z(:)];  % 轨迹位置
% V = [velocity_x(:); velocity_y(:); velocity_z(:)];     % 速度
% a = [acceleration_x(:); acceleration_y(:); acceleration_z(:)]; % 加速度
% else
function [dpt,V,a] = TRACE_Access(t,flag)
% 轨迹规划统一接口
% 输入：flag - 轨迹模式选择
% 输出：dpt - 位置矩阵 [x,y,z]
%       V   - 速度矩阵 [Vx,Vy,Vz]
%       a   - 加速度矩阵 [ax,ay,az]

if flag == 1
    %% x轴 - S曲线轨迹
    % 定义运动参数
    q0_x = 475;     % 初始位置
    q1_x = 425;     % 终止位置
    v0_x = 0;       % 初始速度
    v1_x = 37.5;    % 终止速度
    vmax_x = 50;    % 最大速度
    amax_x = 20;    % 最大加速度
    jmax_x = 60;    % 最大加加速度
    
    % 计算S曲线参数
    para_x = STrajectoryPara(q0_x, q1_x, v0_x, v1_x, vmax_x, amax_x, jmax_x);
    
    % 提取时间参数
    Ta = para_x(1);     % 加速段时间
    Tv = para_x(2);     % 匀速段时间
    Td = para_x(3);     % 减速段时间
    T_total = Ta + Tv + Td;  % 总时间
    
    % 生成时间序列
    t = 0:0.01:T_total;
    
    % 预分配数组
    X = zeros(size(t));
    VX = zeros(size(t));
    aX = zeros(size(t));
    
    % 计算x轴状态
    for i = 1:length(t)
        X(i) = S_position(t(i), para_x(1), para_x(2), para_x(3),para_x(4), para_x(5), para_x(6), para_x(7), para_x(8),para_x(9), para_x(10), para_x(11), para_x(12), para_x(13),para_x(14), para_x(15), para_x(16));
        VX(i) = S_velocity(t(i), para_x(1), para_x(2), para_x(3),para_x(4), para_x(5), para_x(6), para_x(7), para_x(8),para_x(9), para_x(10), para_x(11), para_x(12), para_x(13),para_x(14), para_x(15), para_x(16));
        aX(i) = S_acceleration(t(i), para_x(1), para_x(2), para_x(3), para_x(4), para_x(5), para_x(6), para_x(7), para_x(8),para_x(9), para_x(10), para_x(11), para_x(12), para_x(13), para_x(14), para_x(15), para_x(16));
    end

    %% y轴 - 保持静止
    % 定义静止参数
    q0_y = 0;       % 初始位置 = 终止位置
    q1_y = 0;       % 终止位置
    v0_y = 0;       % 初始速度
    v1_y = 0;       % 终止速度
    vmax_y = 1;     % 任意小正数（避免除零）
    amax_y = 1;     % 任意小正数
    jmax_y = 1;     % 任意小正数
    
    % 计算S曲线参数（结果应为全零运动）
    para_y = STrajectoryPara(q0_y, q1_y, v0_y, v1_y, vmax_y, amax_y, jmax_y);
    
    % 生成静止轨迹
    Y = q0_y * ones(size(t));
    VY = zeros(size(t));
    aY = zeros(size(t));

    %% z轴 - 保持静止（同理）
    q0_z = 980;     % 初始位置 = 终止位置
    q1_z = 980;
    v0_z = 0;
    v1_z = 0;
    vmax_z = 1;
    amax_z = 1;
    jmax_z = 1;
    
    para_z = STrajectoryPara(q0_z, q1_z, v0_z, v1_z, vmax_z, amax_z, jmax_z);
    
    Z = q0_z * ones(size(t));
    VZ = zeros(size(t));
    aZ = zeros(size(t));

    %% 组合输出
    dpt = [X', Y', Z'];
    V = [VX', VY', VZ'];
    a = [aX', aY', aZ'];
    
     
 

  else
    

[K_1,KV_1,Ka_1]=polynomial_v(t,2, 475, 0,0, 325,-90,20);%4-6
[K_2,KV_2,Ka_2]=polynomial_v((t-2),1, 325,-90,20, 225,-120,-10);%6-7
[K_3,KV_3,Ka_3]=polynomial_v((t-3),1, 225,-120,-10, 125,-100,-20);%7-8
[K_4,KV_4,Ka_4]=polynomial_v((t-4),2, 125,-100,-20 , 0,0,0);%8-10
K_5=0;KV_5=0;Ka_5=0;
X=K_1.*(t>=0&t<2)+K_2.*(t>=2&t<3)+K_3.*(t>=3&t<4)+K_4.*(t>=4&t<6)+K_5.*(t>=6&t<=10);
VX=KV_1.*(t>=0&t<2)+KV_2.*(t>=2&t<3)+KV_3.*(t>=3&t<4)+KV_4.*(t>=4&t<6)+KV_5.*(t>=6&t<=10);
aX=Ka_1.*(t>=0&t<2)+Ka_2.*(t>=2&t<3)+Ka_3.*(t>=3&t<4)+Ka_4.*(t>=4&t<6)+Ka_5.*(t>=6&t<=10);



[S_1,SV_1,Sa_1]=polynomial_v(t,2, 0,0,0, 20,15,15);%4-6s
[S_2,SV_2,Sa_2]=polynomial_v((t-2),1, 20,15,15, 45,30,-10);%6-7s
[S_3,SV_3,Sa_3]=polynomial_v((t-3),1, 45,30,-10, 90,80,80);%7-8s
[S_4,SV_4,Sa_4]=polynomial_v((t-4),2, 90,80,80, 225,0,0);%8-10s
S_5=225;SV_5=0;Sa_5=0;
Y=S_1.*(t>=0&t<2)+S_2.*(t>=2&t<3)+S_3.*(t>=3&t<4)+S_4.*(t>=4&t<6)+S_5.*(t>=6&t<=10);
VY=SV_1.*(t>=0&t<2)+SV_2.*(t>=2&t<3)+SV_3.*(t>=3&t<4)+SV_4.*(t>=4&t<6)+SV_5.*(t>=6&t<=10);
aY=Sa_1.*(t>=0&t<2)+Sa_2.*(t>=2&t<3)+Sa_3.*(t>=3&t<4)+Sa_4.*(t>=4&t<6)+Sa_5.*(t>=6&t<=10);

[Z_1,ZV_1,Za_1]=polynomial_v((t-6),4,980,0,0,1300,0,0);
Z_2=980;ZV_2=0;Za_2=0;
Z=Z_2.*(t>=0&t<6)+Z_1.*(t>=6&t<=10);
VZ=ZV_2.*(t>=0&t<6)+ZV_1.*(t>=6&t<=10);
aZ=Za_2.*(t>=0&t<6)+Za_1.*(t>=6&t<=10);

dpt=[X,Y,Z];V=[VX,VY,VZ]; a=[aX,aY,aZ];



end
end

== matlab function new_inkine_2020/MATLAB Function11 ==
  data: t input; dpt output; V output; a output
function [dpt,V,a] = TRACE_Pose_experiment(t)
[K_1,KV_1,Ka_1]=polynomial_v(t,2, 475, 0,0, 325,-90,20);%4-6
[K_2,KV_2,Ka_2]=polynomial_v((t-2),1, 325,-90,20, 225,-120,-10);%6-7
[K_3,KV_3,Ka_3]=polynomial_v((t-3),1, 225,-120,-10, 125,-100,-20);%7-8
[K_4,KV_4,Ka_4]=polynomial_v((t-4),2, 125,-100,-20 , 0,0,0);%8-10
K_5=0;KV_5=0;Ka_5=0;
X=K_1.*(t>=0&t<2)+K_2.*(t>=2&t<3)+K_3.*(t>=3&t<4)+K_4.*(t>=4&t<6)+K_5.*(t>=6&t<=10);
VX=KV_1.*(t>=0&t<2)+KV_2.*(t>=2&t<3)+KV_3.*(t>=3&t<4)+KV_4.*(t>=4&t<6)+KV_5.*(t>=6&t<=10);
aX=Ka_1.*(t>=0&t<2)+Ka_2.*(t>=2&t<3)+Ka_3.*(t>=3&t<4)+Ka_4.*(t>=4&t<6)+Ka_5.*(t>=6&t<=10);



[S_1,SV_1,Sa_1]=polynomial_v(t,2, 0,0,0, 20,15,15);%4-6s
[S_2,SV_2,Sa_2]=polynomial_v((t-2),1, 20,15,15, 45,30,-10);%6-7s
[S_3,SV_3,Sa_3]=polynomial_v((t-3),1, 45,30,-10, 90,80,80);%7-8s
[S_4,SV_4,Sa_4]=polynomial_v((t-4),2, 90,80,80, 225,0,0);%8-10s
S_5=225;SV_5=0;Sa_5=0;
Y=S_1.*(t>=0&t<2)+S_2.*(t>=2&t<3)+S_3.*(t>=3&t<4)+S_4.*(t>=4&t<6)+S_5.*(t>=6&t<=10);
VY=SV_1.*(t>=0&t<2)+SV_2.*(t>=2&t<3)+SV_3.*(t>=3&t<4)+SV_4.*(t>=4&t<6)+SV_5.*(t>=6&t<=10);
aY=Sa_1.*(t>=0&t<2)+Sa_2.*(t>=2&t<3)+Sa_3.*(t>=3&t<4)+Sa_4.*(t>=4&t<6)+Sa_5.*(t>=6&t<=10);

[Z_1,ZV_1,Za_1]=polynomial_v((t-6),4,980,0,0,1300,0,0);
Z_2=980;ZV_2=0;Za_2=0;
Z=Z_2.*(t>=0&t<6)+Z_1.*(t>=6&t<=10);
VZ=ZV_2.*(t>=0&t<6)+ZV_1.*(t>=6&t<=10);
aZ=Za_2.*(t>=0&t<6)+Za_1.*(t>=6&t<=10);

dpt=[X,Y,Z];V=[VX,VY,VZ]; a=[aX,aY,aZ];
end
